simulink model "Project_Final_4_new"  (R2023b)
settings: Solver=VariableStepAuto  StartTime=0.0  StopTime=10.0  RelTol=1e-3
undefined symbols (not defined in the file or in its folder): batData, carData, motorData
libraries: slpidlib x1
settings Model: Creator=stick  LastModifiedBy=stick
settings RTWCC: GPUComputeCapability=5.0

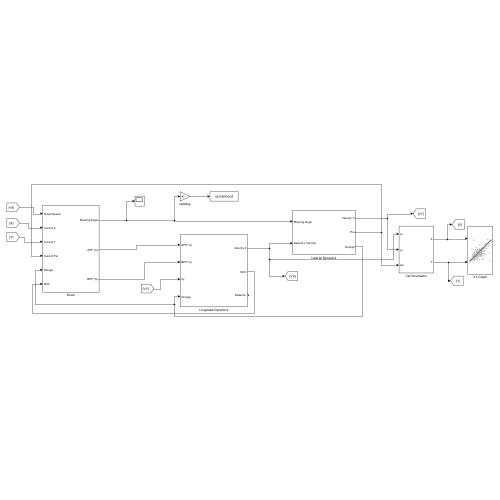
[thumbnail: Simulink's stored preview of the top-level diagram]
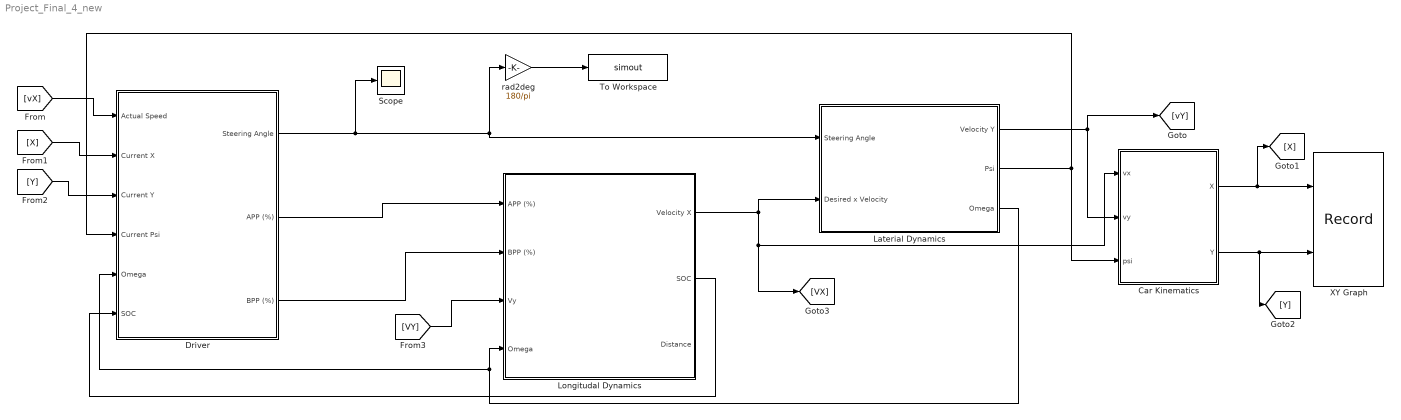
== system Project_Final_4_new ==
  Car Kinematics : Subsystem
  Driver : Subsystem
  Laterial Dynamics : Subsystem
  Longitudal Dynamics : Subsystem
  Scope : Scope
  To Workspace : ToWorkspace  VariableName=simout  SaveFormat=Timeseries  SampleTime=-1
  XY Graph : Record  FileSettingsInternal="{\"entries\":[{\"content\":{\"excelSettings\":{\"content\":{},\"type\":\"Streamout.ExcelSettings\"}},\"type\":\"Streamout.FileSettingStorage\",\"uuid\":\"\"}],\"packageUris\":[\"http:\\/\\/schema.mathworks.com\\/mf0\\/streamout_blocks\\/R2020a\"],\"version\":\"1.0\"}"  Layout=[1 1]  SignalsInternal="{\"entries\":[{\"content\":{\"signals\":[{\"content\":{\"blockPath\":[],\"dimensions\":[1],\"domain\":\"\",\"lineColor\":\"#d95319\",\"plots\":[ 1 ],\"port\":1,\"signalID\":1,\"signalName\":\"Car Kinematics:1\"},\"type\":\"RecordBlkView.Signal\",\"uuid\":\"\"},{\"content\":{\"blockPath\":[],\"dimensions\":[1],\"domain\":\"\",\"lineColor\":\"#edb120\",\"plots\":[ 1 ],\"port\":2,\"signalID\":2,\"signalName\":\"Car Kinematics:2\"},\"type\":\"RecordBlkView.Signal\",\"uuid\":\"\"}]},\"type\":\"RecordBlkView.InputSignals\",\"uuid\":\"\"}],\"packageUris\":[\"http:\\/\\/schema.mathworks.com\\/mf0\\/streamout_blocks\\/R2020a\"],\"version\":\"1.0\"}"  VisualizationBindings="{\"xyplotplugin\":{\"info\":[{\"series\":[{\"bindingParametersList\":[{\"parameter\":\"X-Axis\",\"signalID\":1,\"signalName\":\"Car Kinematics:1\"},{\"parameter\":\"Y-Axis\",\"signalID\":2,\"signalName\":\"Car Kinematics:2\"}],\"seriesID\":0}],\"subplotID\":1}]}}"  CompatibilityTag=XY  st=-1
  rad2deg : Gain  Gain=180/pi
  wires:
  [VY] -> Longitudal Dynamics/3(Vy)
  Driver/2(APP (%)) -> Longitudal Dynamics/1(APP (%))
  Driver/3(BPP (%)) -> Longitudal Dynamics/2(BPP (%))
  Laterial Dynamics/1(Velocity Y) -> [vY], Car Kinematics/2(vy)
  Longitudal Dynamics/1(Velocity X) -> [VX], Car Kinematics/1(vx), Laterial Dynamics/2(Desired x Velocity)
  Laterial Dynamics/2(Psi) -> Driver/4(Current Psi), Car Kinematics/3(psi)
  Laterial Dynamics/3(Omega) -> Longitudal Dynamics/4(Omega), Driver/5(Omega)
  Longitudal Dynamics/2(SOC) -> Driver/6(SOC)
  Driver/1(Steering Angle) -> Scope/1, rad2deg/1, Laterial Dynamics/1(Steering Angle)
  Car Kinematics/1(X) -> [X], XY Graph/1
  Car Kinematics/2(Y) -> [Y], XY Graph/2
  rad2deg/1 -> To Workspace/1
  [vX] -> Driver/1(Actual Speed)
  [X] -> Driver/2(Current X)
  [Y] -> Driver/3(Current Y)

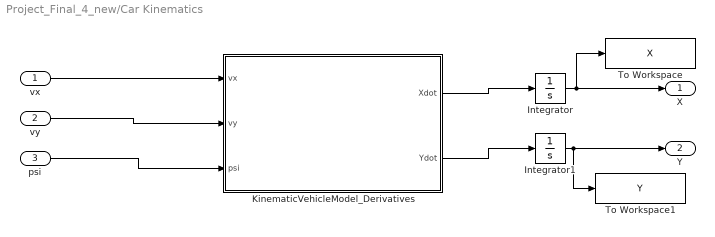
== system Project_Final_4_new/Car Kinematics ==
  vx : Inport
  vy : Inport  Port=2
  psi : Inport  Port=3
  Integrator : Integrator  InitialCondition=carData.init.X0
  Integrator1 : Integrator  InitialCondition=carData.init.Y0
  KinematicVehicleModel_Derivatives : MATLAB Function  TreatAsAtomicUnit=on
  To Workspace : ToWorkspace  VariableName=X  SaveFormat=Timeseries  SampleTime=-1
  To Workspace1 : ToWorkspace  VariableName=Y  SaveFormat=Timeseries  SampleTime=-1
  X : Outport
  Y : Outport  Port=2
  wires:
  Integrator1/1 -> To Workspace1/1, Y/1
  vy/1 -> KinematicVehicleModel_Derivatives/2(vy)
  vx/1 -> KinematicVehicleModel_Derivatives/1(vx)
  KinematicVehicleModel_Derivatives/2(Ydot) -> Integrator1/1
  psi/1 -> KinematicVehicleModel_Derivatives/3(psi)
  Integrator/1 -> To Workspace/1, X/1
  KinematicVehicleModel_Derivatives/1(Xdot) -> Integrator/1

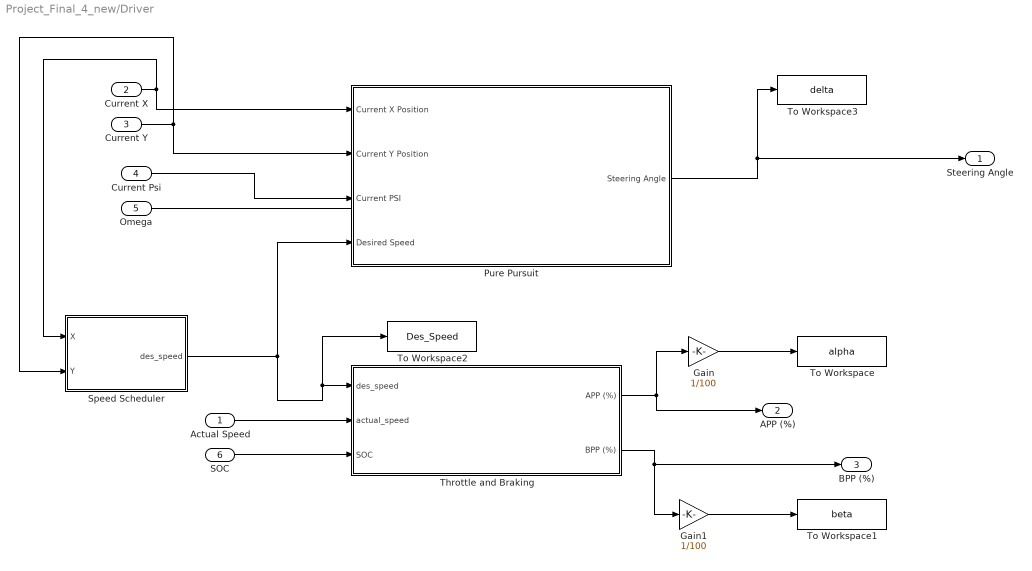
== system Project_Final_4_new/Driver ==
  Actual Speed : Inport
  Current X : Inport  Port=2
  Current Y : Inport  Port=3
  Current Psi : Inport  Port=4
  Omega : Inport  Port=5
  SOC : Inport  Port=6
  Gain : Gain  Gain=1/100
  Gain1 : Gain  Gain=1/100
  Pure Pursuit : Subsystem
  Speed Scheduler : MATLAB Function  TreatAsAtomicUnit=on
  Throttle and Braking : Subsystem
  To Workspace : ToWorkspace  VariableName=alpha  SaveFormat=Timeseries  SampleTime=-1
  To Workspace1 : ToWorkspace  VariableName=beta  SaveFormat=Timeseries  SampleTime=-1
  To Workspace2 : ToWorkspace  VariableName=Des_Speed  SaveFormat=Timeseries  SampleTime=-1
  To Workspace3 : ToWorkspace  VariableName=delta  SaveFormat=Timeseries  SampleTime=-1
  Steering Angle : Outport
  APP (%) : Outport  Port=2
  BPP (%) : Outport  Port=3
  wires:
  Throttle and Braking/1(APP (%)) -> APP (%)/1, Gain/1
  Throttle and Braking/2(BPP (%)) -> BPP (%)/1, Gain1/1
  Speed Scheduler/1(des_speed) -> To Workspace2/1, Throttle and Braking/1(des_speed), Pure Pursuit/4(Desired Speed)
  Pure Pursuit/1(Steering Angle) -> Steering Angle/1, To Workspace3/1
  Gain/1 -> To Workspace/1
  Gain1/1 -> To Workspace1/1
  Actual Speed/1 -> Throttle and Braking/2(actual_speed)
  SOC/1 -> Throttle and Braking/3(SOC)
  Current Psi/1 -> Pure Pursuit/3(Current PSI)
  Omega/1 -> ?
  Current X/1 -> Speed Scheduler/1(X), Pure Pursuit/1(Current X Position)
  Current Y/1 -> Speed Scheduler/2(Y), Pure Pursuit/2(Current Y Position)

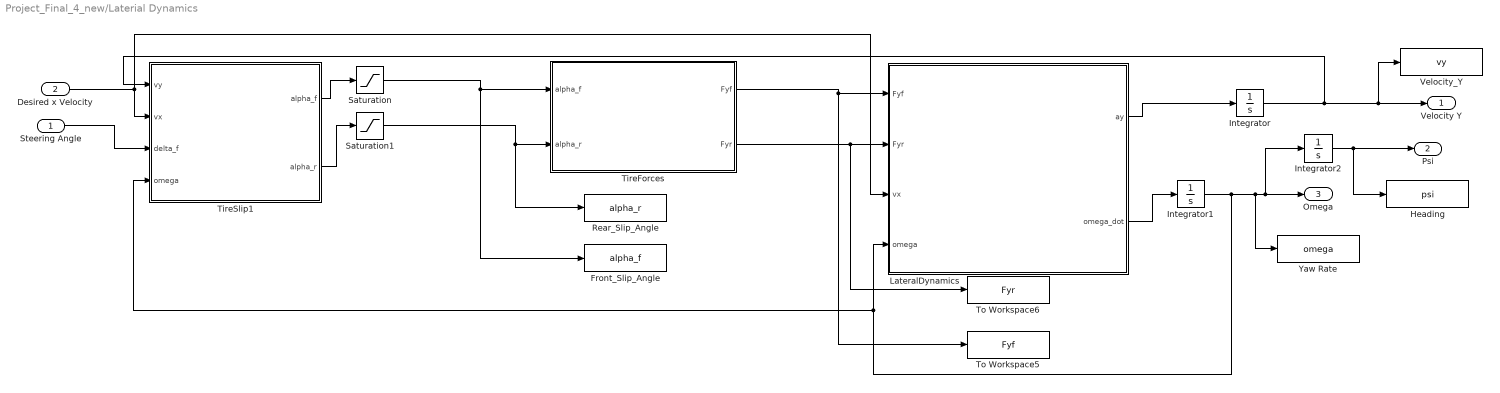
== system Project_Final_4_new/Laterial Dynamics ==
  Steering Angle : Inport
  Desired x Velocity : Inport  Port=2
  Front_Slip_Angle : ToWorkspace  VariableName=alpha_f  SaveFormat=Timeseries  SampleTime=-1
  Heading : ToWorkspace  VariableName=psi  SaveFormat=Timeseries  SampleTime=-1
  Integrator : Integrator  InitialCondition=carData.init.vy0
  Integrator1 : Integrator  InitialCondition=carData.init.omega0
  Integrator2 : Integrator  InitialCondition=carData.init.psi0  WrappedStateUpperValue=2*pi  WrappedStateLowerValue=0
  LateralDynamics : MATLAB Function  TreatAsAtomicUnit=on
  Rear_Slip_Angle : ToWorkspace  VariableName=alpha_r  SaveFormat=Timeseries  SampleTime=-1
  Saturation : Saturate  UpperLimit=carData.maxAlpha  LowerLimit=-carData.maxAlpha
  Saturation1 : Saturate  UpperLimit=carData.maxAlpha  LowerLimit=-carData.maxAlpha
  TireForces : MATLAB Function  TreatAsAtomicUnit=on
  TireSlip1 : MATLAB Function  TreatAsAtomicUnit=on
  To Workspace5 : ToWorkspace  VariableName=Fyf  SaveFormat=Timeseries  SampleTime=-1
  To Workspace6 : ToWorkspace  VariableName=Fyr  SaveFormat=Timeseries  SampleTime=-1
  Velocity_Y : ToWorkspace  VariableName=vy  SaveFormat=Timeseries  SampleTime=-1
  Yaw Rate : ToWorkspace  VariableName=omega  SaveFormat=Timeseries  SampleTime=-1
  Velocity Y : Outport
  Psi : Outport  Port=2
  Omega : Outport  Port=3
  wires:
  TireSlip1/2(alpha_r) -> Saturation1/1
  Integrator1/1 -> Omega/1, Integrator2/1, Yaw Rate/1, LateralDynamics/4(omega), TireSlip1/4(omega)
  LateralDynamics/1(ay) -> Integrator/1
  Saturation/1 -> Front_Slip_Angle/1, TireForces/1(alpha_f)
  TireForces/2(Fyr) -> LateralDynamics/2(Fyr), To Workspace6/1
  Steering Angle/1 -> TireSlip1/3(delta_f)
  LateralDynamics/2(omega_dot) -> Integrator1/1
  Desired x Velocity/1 -> TireSlip1/2(vx), LateralDynamics/3(vx)
  TireSlip1/1(alpha_f) -> Saturation/1
  Integrator2/1 -> Psi/1, Heading/1
  TireForces/1(Fyf) -> LateralDynamics/1(Fyf), To Workspace5/1
  Integrator/1 -> TireSlip1/1(vy), Velocity Y/1, Velocity_Y/1
  Saturation1/1 -> TireForces/2(alpha_r), Rear_Slip_Angle/1

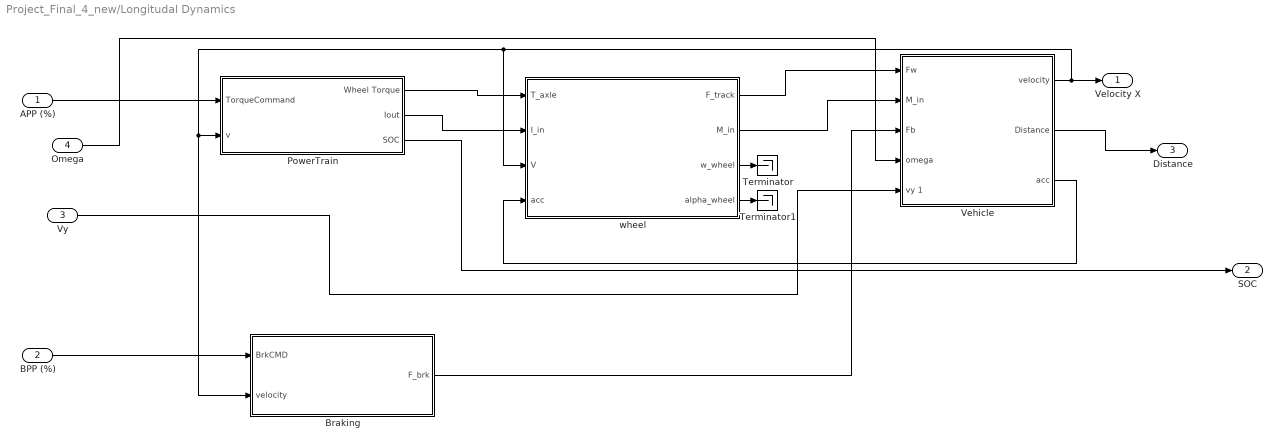
== system Project_Final_4_new/Longitudal Dynamics ==
  APP (%) : Inport
  BPP (%) : Inport  Port=2
  Vy : Inport  Port=3
  Omega : Inport  Port=4
  Braking : Subsystem
  PowerTrain : Subsystem
  Terminator : Terminator
  Terminator1 : Terminator
  Vehicle : Subsystem
  "wheel " : Subsystem
  Velocity X : Outport
  SOC : Outport  Port=2
  "Distance " : Outport  Port=3
  wires:
  Vehicle/1("velocity ") -> Velocity X/1, Braking/2("velocity "), PowerTrain/2(v), "wheel "/3(V)
  "wheel "/3(w_wheel) -> Terminator/1
  "wheel "/4(alpha_wheel) -> Terminator1/1
  APP (%)/1 -> PowerTrain/1(TorqueCommand)
  Vehicle/3(acc) -> "wheel "/4(acc)
  "wheel "/2(M_in) -> Vehicle/2("M_in ")
  "wheel "/1(F_track) -> Vehicle/1("Fw ")
  Vy/1 -> Vehicle/5(vy 1)
  Braking/1("F_brk ") -> Vehicle/3("Fb ")
  PowerTrain/2(Iout) -> "wheel "/2(I_in)
  PowerTrain/1(Wheel Torque) -> "wheel "/1(T_axle)
  Omega/1 -> Vehicle/4(omega)
  BPP (%)/1 -> Braking/1("BrkCMD ")
  PowerTrain/3(SOC) -> SOC/1
  Vehicle/2("Distance ") -> "Distance "/1

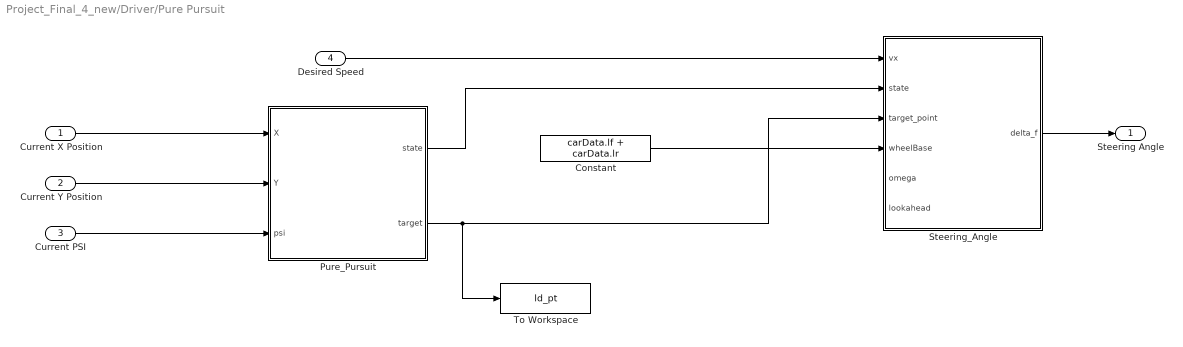
== system Project_Final_4_new/Driver/Pure Pursuit ==
  Current X Position : Inport
  Current Y Position : Inport  Port=2
  Current PSI : Inport  Port=3
  Desired Speed : Inport  Port=4
  Constant : Constant  Value=carData.lf + carData.lr
  Pure_Pursuit : MATLAB Function  TreatAsAtomicUnit=on
  Steering_Angle : MATLAB Function  TreatAsAtomicUnit=on
  To Workspace : ToWorkspace  VariableName=ld_pt  SaveFormat=Timeseries  SampleTime=-1
  Steering Angle : Outport
  wires:
  Constant/1 -> Steering_Angle/4(wheelBase)
  Steering_Angle/1(delta_f) -> Steering Angle/1
  Pure_Pursuit/2(target) -> Steering_Angle/3(target_point), To Workspace/1
  Pure_Pursuit/1(state) -> Steering_Angle/2(state)
  Desired Speed/1 -> Steering_Angle/1(vx)
  Current PSI/1 -> Pure_Pursuit/3(psi)
  Current Y Position/1 -> Pure_Pursuit/2(Y)
  Current X Position/1 -> Pure_Pursuit/1(X)

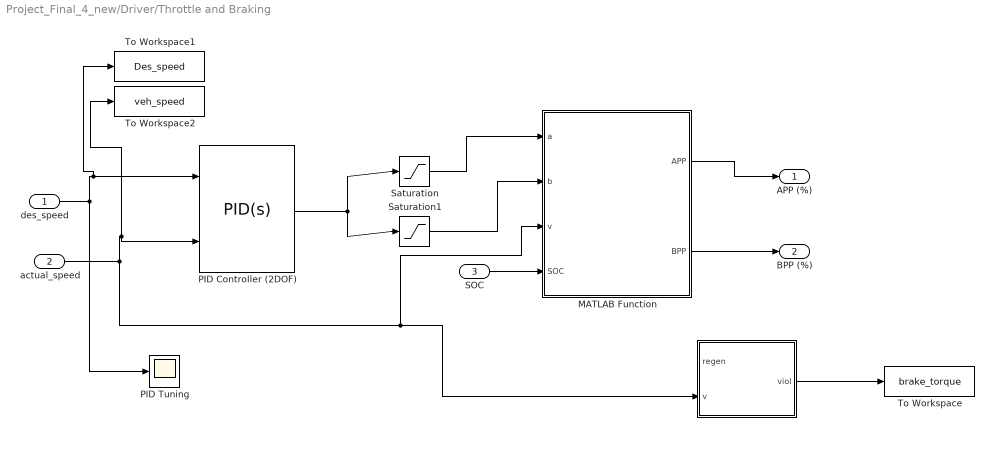
== system Project_Final_4_new/Driver/Throttle and Braking ==
  des_speed : Inport
  actual_speed : Inport  Port=2
  SOC : Inport  Port=3
  "  " : MATLAB Function  TreatAsAtomicUnit=on
  MATLAB Function : MATLAB Function  TreatAsAtomicUnit=on
  PID Controller (2DOF) : slpidlib/PID Controller (2DOF)  Controller=PID  Form=Parallel  TimeDomain=Continuous-time  UseExternalTs=off  SampleTime=-1  IntegratorMethod=Forward Euler  FilterMethod=Forward Euler  ControllerParametersSource=internal  P=1  I=1  UseKiTs=off  D=0  N=100  UseFilter=on  b=1  c=1  TunerSelectOption=Transfer Function Based (PID Tuner App)  InitialConditionSource=internal  InitialConditionForIntegrator=0  InitialConditionForFilter=0  DifferentiatorICPrevScaledInput=0  ExternalReset=none  TrackingMode=off  Kt=1  LimitOutput=off  SatLimitsSource=internal  UpperSaturationLimit=inf  LowerSaturationLimit=-inf  LinearizeAsGain=on  AntiWindupMode=none  Kb=1  LimitIntegrator=off  UpperIntegratorSaturationLimit=inf  LowerIntegratorSaturationLimit=-inf  POutMin=[]  POutMax=[]  IOutMin=[]  IOutMax=[]  DOutMin=[]  DOutMax=[]  NOutMin=[]  NOutMax=[]  bOutMin=[]  bOutMax=[]  cOutMin=[]  cOutMax=[]  SumOutMin=[]  SumOutMax=[]  SaturationOutMin=[]  SaturationOutMax=[]  PParamMin=[]  PParamMax=[]  IParamMin=[]  IParamMax=[]  DParamMin=[]  DParamMax=[]  NParamMin=[]  NParamMax=[]  bParamMin=[]  bParamMax=[]  cParamMin=[]  cParamMax=[]  KbParamMin=[]  KbParamMax=[]  KtParamMin=[]  KtParamMax=[]  KbOutMin=[]  KbOutMax=[]  KtOutMin=[]  KtOutMax=[]  IntegratorOutMin=[]  IntegratorOutMax=[]  FilterOutMin=[]  FilterOutMax=[]  SumI1OutMin=[]  SumI1OutMax=[]  SumI2OutMin=[]  SumI2OutMax=[]  SumI3OutMin=[]  SumI3OutMax=[]  SumI4OutMin=[]  SumI4OutMax=[]  SumDOutMin=[]  SumDOutMax=[]  Sum1OutMin=[]  Sum1OutMax=[]  Sum2OutMin=[]  Sum2OutMax=[]  Sum3OutMin=[]  Sum3OutMax=[]  DifferentiatorOutMin=[]  DifferentiatorOutMax=[]  FilterDiffOutCoefMin=[]  FilterDiffOutCoefMax=[]  ReciprocalOutMin=[]  ReciprocalOutMax=[]  SumDenOutMin=[]  SumDenOutMax=[]  SumNumOutMin=[]  SumNumOutMax=[]  DivideOutMin=[]  DivideOutMax=[]  UdiffTsProdOutMin=[]  UdiffTsProdOutMax=[]  NTsProdOutMin=[]  NTsProdOutMax=[]  UintegralTsProdOutMin=[]  UintegralTsProdOutMax=[]  UngainTsProdOutMin=[]  UngainTsProdOutMax=[]  ClampingZeroOutDataTypeStr=Inherit: Inherit via back propagation  ClampingZeroOutMin=[]  ClampingZeroOutMax=[]  FilterDenConstantOutDataTypeStr=Inherit: Inherit via back propagation  FilterDenConstantOutMin=[]  FilterDenConstantOutMax=[]  PCopyOutDataTypeStr=Inherit: Inherit via back propagation  PCopyOutMin=[]  PCopyOutMax=[]  NCopyOutDataTypeStr=Inherit: Inherit via back propagation  NCopyOutMin=[]  NCopyOutMax=[]  IntegratorContinuousStateAttributes=''  IntegratorStateMustResolveToSignalObject=off  IntegratorRTWStateStorageClass=Auto  FilterContinuousStateAttributes=''  FilterStateMustResolveToSignalObject=off  FilterRTWStateStorageClass=Auto  ParallelPVariant=InternalParameters  IdealPVariant=Disabled  IVariant=InternalParameters  DVariant=InternalParameters  bVariant=InternalParameters  cVariant=InternalParameters  IntegratorVariant=Continuous  SatVariant=Disabled  AWVariant=Passthrough  PCopyVariant=Disabled  TRVariant=Disabled  FdbkBlocksVariant=Forward  IdealPFdbkVariant=Disabled  SatFdbkVariant=Disabled  DerivativeFilterVariant=ContFilter  NVariant=InternalParameters  NCopyVariant=Disabled  FilterICVariant=InternalICsFilter  IntegratorICVariant=InternalICs  ExternalResetVariant=Disabled  TRSumVariant=Passthrough  SumFdbkVariant=Disabled  SumVariant=Sum_PID  TsampFilterVariant=InternalTs  TsampNgainVariant=Passthrough  TsampIntegralVariant=Disabled_SignalSpec  ExternalSaturationOutDataTypeStr=Inherit: Same as second input
  PID Tuning : Scope
  Saturation : Saturate  UpperLimit=1  LowerLimit=0
  Saturation1 : Saturate  UpperLimit=0  LowerLimit=-1
  To Workspace : ToWorkspace  VariableName=brake_torque  SaveFormat=Timeseries  SampleTime=-1
  To Workspace1 : ToWorkspace  VariableName=Des_speed  SaveFormat=Timeseries  SampleTime=-1
  To Workspace2 : ToWorkspace  VariableName=veh_speed  SaveFormat=Timeseries  SampleTime=-1
  APP (%) : Outport
  BPP (%) : Outport  Port=2
  wires:
  des_speed/1 -> PID Tuning/1, To Workspace1/1, PID Controller (2DOF)/1
  PID Controller (2DOF)/1 -> Saturation1/1, Saturation/1
  "  "/1(viol) -> To Workspace/1
  actual_speed/1 -> MATLAB Function/3(v), "  "/2(v), To Workspace2/1, PID Controller (2DOF)/2
  SOC/1 -> MATLAB Function/4(SOC)
  MATLAB Function/2(BPP) -> BPP (%)/1
  MATLAB Function/1(APP) -> APP (%)/1
  Saturation/1 -> MATLAB Function/1(a)
  Saturation1/1 -> MATLAB Function/2(b)

== system Project_Final_4_new/Longitudal Dynamics/Braking ==
  "BrkCMD " : Inport
  "velocity " : Inport  Port=2
  Gain1 : Gain  Gain=1.09
  MATLAB Function : MATLAB Function  TreatAsAtomicUnit=on
  "F_brk " : Outport  VectorParamsAs1DForOutWhenUnconnected=off
  wires:
  "BrkCMD "/1 -> Gain1/1
  Gain1/1 -> MATLAB Function/1(u)
  MATLAB Function/1(y) -> "F_brk "/1
  "velocity "/1 -> MATLAB Function/2(v)

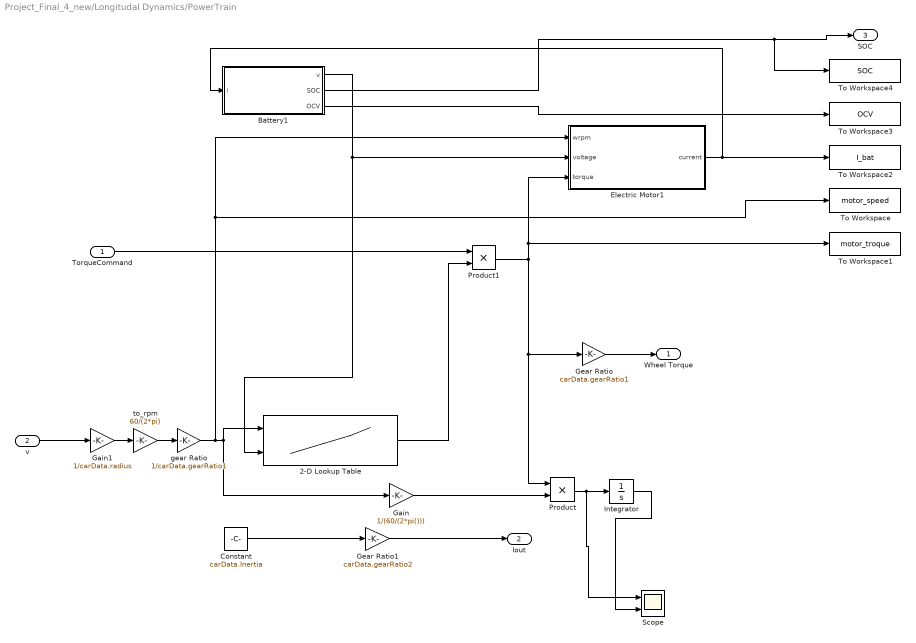
== system Project_Final_4_new/Longitudal Dynamics/PowerTrain ==
  TorqueCommand : Inport
  v : Inport  Port=2
  2-D Lookup Table : Lookup_n-D  BreakpointsForDimension1=motorData.vbus  BreakpointsForDimension2=motorData.rpm  Table=motorData.maxtorque  InternalRulePriority=Speed  RndMeth=Simplest
      settings: InputPortMap=u0,u1
  Battery1 : Subsystem
  Constant : Constant  Value=carData.Inertia
  Electric Motor1 : Subsystem
  Gain : Gain  Gain=1/(60/(2*pi()))
  Gain1 : Gain  Gain=1/carData.radius
  Gear Ratio : Gain  Gain=carData.gearRatio1
  Gear Ratio1 : Gain  Gain=carData.gearRatio2
  Integrator : Integrator
  Product : Product
  Product1 : Product
  Scope : Scope  NumInputPorts=2
  To Workspace : ToWorkspace  VariableName=motor_speed  SaveFormat=Structure With Time  SampleTime=-1
  To Workspace1 : ToWorkspace  VariableName=motor_troque  SaveFormat=Structure With Time  SampleTime=-1
  To Workspace2 : ToWorkspace  VariableName=I_bat  SaveFormat=Structure With Time  SampleTime=-1
  To Workspace3 : ToWorkspace  VariableName=OCV  SaveFormat=Structure With Time  SampleTime=-1
  To Workspace4 : ToWorkspace  VariableName=SOC  SaveFormat=Structure With Time  SampleTime=-1
  gear Ratio : Gain  Gain=1/carData.gearRatio1
  to_rpm : Gain  Gain=60/(2*pi)
  Wheel Torque : Outport
  Iout : Outport  Port=2
  SOC : Outport  Port=3
  wires:
  TorqueCommand/1 -> Product1/1
  Constant/1 -> Gear Ratio1/1
  v/1 -> Gain1/1
  Gain1/1 -> to_rpm/1
  2-D Lookup Table/1 -> Product1/2
  Product1/1 -> Product/1, Gear Ratio/1, Electric Motor1/3(torque), To Workspace1/1
  to_rpm/1 -> gear Ratio/1
  gear Ratio/1 -> Electric Motor1/1(wrpm), To Workspace/1, Gain/1, 2-D Lookup Table/1
  Gear Ratio/1 -> Wheel Torque/1
  Product/1 -> Scope/1, Integrator/1
  Integrator/1 -> Scope/2
  Gain/1 -> Product/2
  Battery1/1(v) -> 2-D Lookup Table/2, Electric Motor1/2(voltage)
  Electric Motor1/1(current) -> To Workspace2/1, Battery1/1(i)
  Gear Ratio1/1 -> Iout/1
  Battery1/2(SOC) -> To Workspace4/1, SOC/1
  Battery1/3(OCV) -> To Workspace3/1

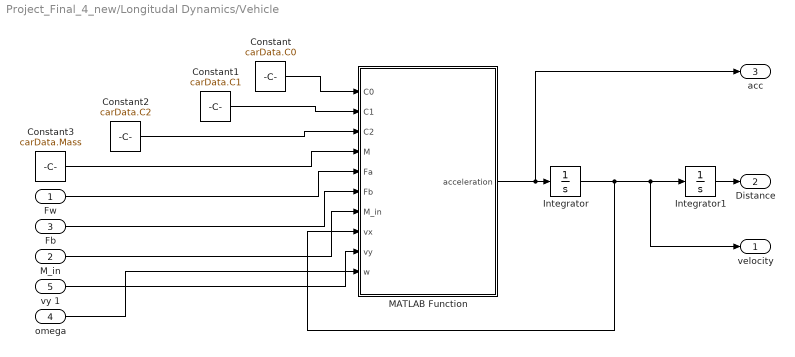
== system Project_Final_4_new/Longitudal Dynamics/Vehicle ==
  "Fw " : Inport
  "M_in " : Inport  Port=2
  "Fb " : Inport  Port=3
  omega : Inport  Port=4
  vy 1 : Inport  Port=5
  Constant : Constant  Value=carData.C0
  Constant1 : Constant  Value=carData.C1
  Constant2 : Constant  Value=carData.C2
  Constant3 : Constant  Value=carData.Mass
  Integrator : Integrator  LimitOutput=on  LowerSaturationLimit=0
  Integrator1 : Integrator
  MATLAB Function : MATLAB Function  TreatAsAtomicUnit=on
  "velocity " : Outport  VectorParamsAs1DForOutWhenUnconnected=off
  "Distance " : Outport  Port=2  VectorParamsAs1DForOutWhenUnconnected=off
  acc : Outport  Port=3
  wires:
  Constant1/1 -> MATLAB Function/2(C1)
  Constant/1 -> MATLAB Function/1(C0)
  MATLAB Function/1(acceleration) -> acc/1, Integrator/1
  Constant2/1 -> MATLAB Function/3(C2)
  Constant3/1 -> MATLAB Function/4(M)
  "Fw "/1 -> MATLAB Function/5(Fa)
  "Fb "/1 -> MATLAB Function/6(Fb)
  Integrator/1 -> MATLAB Function/8(vx), "velocity "/1, Integrator1/1
  Integrator1/1 -> "Distance "/1
  "M_in "/1 -> MATLAB Function/7(M_in)
  omega/1 -> MATLAB Function/10(w)
  vy 1/1 -> MATLAB Function/9(vy)

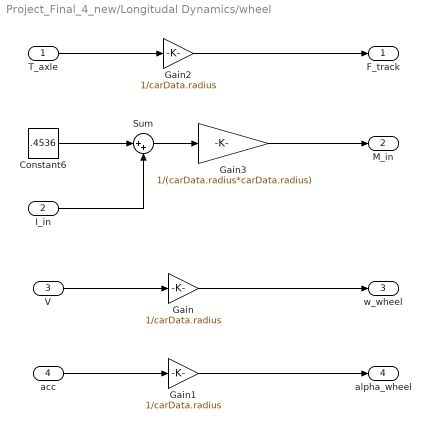
== system Project_Final_4_new/Longitudal Dynamics/wheel  ==
  T_axle : Inport
  I_in : Inport  Port=2
  V : Inport  Port=3
  acc : Inport  Port=4
  Constant6 : Constant  Value=.4536
  Gain : Gain  Gain=1/carData.radius
  Gain1 : Gain  Gain=1/carData.radius
  Gain2 : Gain  Gain=1/carData.radius
  Gain3 : Gain  Gain=1/(carData.radius*carData.radius)
  Sum : Sum  Inputs=|++
  F_track : Outport
  M_in : Outport  Port=2
  w_wheel : Outport  Port=3
  alpha_wheel : Outport  Port=4
  wires:
  Gain/1 -> w_wheel/1
  V/1 -> Gain/1
  acc/1 -> Gain1/1
  Gain1/1 -> alpha_wheel/1
  T_axle/1 -> Gain2/1
  Gain2/1 -> F_track/1
  Gain3/1 -> M_in/1
  Constant6/1 -> Sum/1
  I_in/1 -> Sum/2
  Sum/1 -> Gain3/1

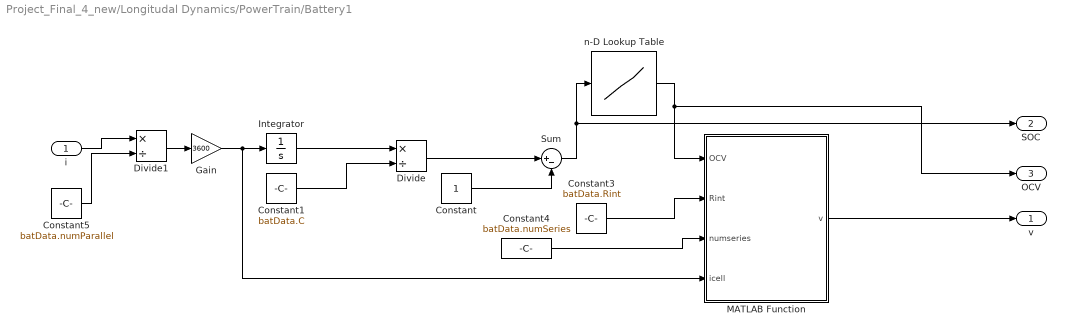
== system Project_Final_4_new/Longitudal Dynamics/PowerTrain/Battery1 ==
  i : Inport
  Constant : Constant
  Constant1 : Constant  Value=batData.C
  Constant3 : Constant  Value=batData.Rint
  Constant4 : Constant  Value=batData.numSeries
  Constant5 : Constant  Value=batData.numParallel
  Divide : Product  Inputs=*/
  Divide1 : Product  Inputs=*/
  Gain : Gain  Gain=3600
  Integrator : Integrator
  MATLAB Function : MATLAB Function  TreatAsAtomicUnit=on
  Sum : Sum  Inputs=|+-
  n-D Lookup Table : Lookup_n-D  NumberOfTableDimensions=1  BreakpointsForDimension1=batData.SOC  BreakpointsForDimension3=[5, 7]  Table=batData.OCV  InternalRulePriority=Speed  RndMeth=Simplest
  v : Outport
  SOC : Outport  Port=2
  OCV : Outport  Port=3
  wires:
  Constant/1 -> Sum/2
  Integrator/1 -> Divide/1
  Divide/1 -> Sum/1
  Constant1/1 -> Divide/2
  MATLAB Function/1(v) -> v/1
  Constant4/1 -> MATLAB Function/3(numseries)
  Divide1/1 -> Gain/1
  Constant5/1 -> Divide1/2
  i/1 -> Divide1/1
  Constant3/1 -> MATLAB Function/2(Rint)
  Sum/1 -> SOC/1, n-D Lookup Table/1
  n-D Lookup Table/1 -> OCV/1, MATLAB Function/1(OCV)
  Gain/1 -> MATLAB Function/4(icell), Integrator/1

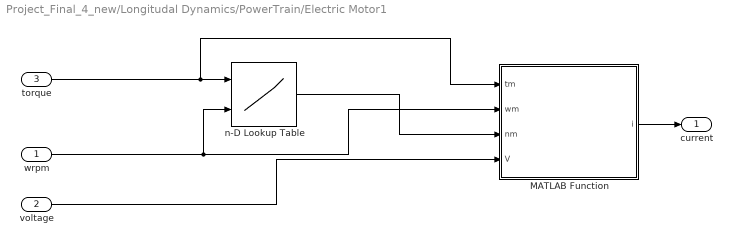
== system Project_Final_4_new/Longitudal Dynamics/PowerTrain/Electric Motor1 ==
  wrpm : Inport
  voltage : Inport  Port=2
  torque : Inport  Port=3
  MATLAB Function : MATLAB Function  TreatAsAtomicUnit=on
  n-D Lookup Table : Lookup_n-D  BreakpointsForDimension1=motorData.eta_torque  BreakpointsForDimension2=motorData.eta_speed  BreakpointsForDimension3=[5, 7]  Table=motorData.eta_val  InternalRulePriority=Speed  RndMeth=Simplest
      settings: InputPortMap=u0,u1
  current : Outport
  wires:
  torque/1 -> MATLAB Function/1(tm), n-D Lookup Table/1
  wrpm/1 -> MATLAB Function/2(wm), n-D Lookup Table/2
  n-D Lookup Table/1 -> MATLAB Function/3(nm)
  MATLAB Function/1(i) -> current/1
  voltage/1 -> MATLAB Function/4(V)

== matlab function Project_Final_4_new/Driver/Pure Pursuit/Pure_Pursuit ==
  data: state output; target output; X input; Y input; psi input
function [state,target] = fcn(X,Y, psi)

% creating a racetrack
% variables

x_i = [0];
y_i = [0];
x_o = [0];
x_p =[0];
y_p = [7.5];
y_o = [15];
radius = 200;
radius2 = 185;
center_right = [900,-200];
center_left = [0,-200];
theta = linspace(0,pi,1000);

% loop to obtain all values

for i = 1:900;
    j_i = 0;
    j_o = 7.5;
    x_p = [x_p, i];
    y_p = [y_p,j_i];
    x_i = [x_i, i];
    x_o = [x_o,i];
    y_o = [y_o,j_o];
    y_i = [y_i,j_i];
end

for i = 1:length(theta);
    x_o = [x_o, center_right(1)+radius*sin(theta(i))];
    x_i = [x_i, center_right(1)+radius2*sin(theta(i))];
    x_p = [x_p, center_right(1)+radius2*sin(theta(i))];
    y_p = [y_p, 15 + center_right(2)+radius*cos(theta(i))];
    y_o = [y_o, 15 + center_right(2)+radius*cos(theta(i))];
    y_i = [y_i, 15 + center_right(2)+radius2*cos(theta(i))];
end 

for i = 1:900;
    x_o = [x_o,900-i];
    x_i = [x_i,900-i];
    x_p = [x_p, 900-i];
    y_p = [y_p,-377.5];
    y_o = [y_o, -385];
    y_i = [y_i,-370];
end 

for i = 1:length(theta);
    x_o = [x_o, center_left(1)-radius*sin(theta(i))];
    x_i = [x_i, center_left(1)-radius2*sin(theta(i))];
    x_p = [x_p, center_left(1)-radius2*sin(theta(i))];
    y_p = [y_p, 15 + center_left(2)-radius*cos(theta(i))];
    y_o = [y_o, 15 + center_left(2)-radius*cos(theta(i))];
    y_i = [y_i, 15 + center_left(2)-radius2*cos(theta(i))];
end

waypoints_x = x_p;
waypoints_y = y_p;

% plotting racetrack
%plot(x_i, y_i)
%axis([-100 1000 -400 25])
%hold on
%plot(x_o,y_o)
%hold off

% code for plotting animated moving car
%variables for finding path to plot

x_p = [0];
y_p = [];
center_rightpath = [0,-192.5];
center_leftpath = [900,-192.5];
radius_path = -192.5; 

for i = 1:900;
    x_p = [x_p, i];
    y_p = [y_p,7.5];
end

for i = 1:length(theta);
    x_p = [x_p, center_leftpath(1)-radius_path*sin(theta(i))];
    y_p = [y_p, 7.5 + center_leftpath(2)-radius_path*cos(theta(i))];
end 

for i = 1:900;
    x_p = [x_p,900-i];
    y_p = [y_p,-377.5];
end 

for i = 1:length(theta);
    x_p = [x_p, center_rightpath(1)+radius_path*sin(theta(i))];
    y_p = [y_p, 7.5 + center_rightpath(2)+radius_path*cos(theta(i))];

end   
waypoints_y;
waypoints_x;

dist = zeros(1, numel(waypoints_x));

for i = 1:numel(waypoints_x)
    dist(i) = sqrt((waypoints_x(i) - X)^2 + (waypoints_y(i) - Y)^2);

end

[~, index] = min(dist);

target_psi = atan2(waypoints_y(index) - Y, waypoints_x(index) - X);


state =[X,Y,psi];

target = [waypoints_x(index), waypoints_y(index), target_psi];

== matlab function Project_Final_4_new/Driver/Pure Pursuit/Steering_Angle ==
  data: vx input; delta_f output; state input; target_point input; wheelBase input; omega input; lookahead input

function delta_f = latControl(vx, state, target_point, wheelBase, omega, lookahead)

current_X = state(1);
current_Y = state(2);
current_psi = state(3);

targ_X = target_point(1);
targ_Y = target_point(2);
tar_psi = target_point(3);

alpha = atan2(targ_Y-current_Y,targ_X - current_X)-current_psi;
psi_dot_d = (2*wheelbase*sin(alpha))/lookahead;
delta_f = atan(psi_dot_d);

== matlab function Project_Final_4_new/Driver/Throttle and Braking/MATLAB Function ==
  data: a input; b input; APP output; v input; SOC input; BPP output
function [APP,BPP] = fcn(a,b,v, SOC)
v = v;
SOC = SOC;
if a>0
    APP=a;
    BPP=0;
elseif b<0
    APP=0;
    BPP=b;
else
    APP=0;
    BPP=0;
end

== matlab function Project_Final_4_new/Laterial Dynamics/TireSlip1 ==
  data: vy input; alpha_f output; vx input; delta_f input; omega input; alpha_r output
function [alpha_f, alpha_r] = fnc(vy, vx, delta_f, omega)

    if abs(vx) > 0.1
        alpha_f = delta_f - (vy + omega *1) / vx;
        alpha_r = - (vy - omega * 1.5) / vx;
    else
        alpha_f = 0;
        alpha_r = 0;
    end

end

== matlab function Project_Final_4_new/Laterial Dynamics/LateralDynamics ==
  data: Fyf input; ay output; Fyr input; vx input; omega input; omega_dot output
function [ay, omega_dot] = fcn(Fyf, Fyr, vx, omega)

    Fy = Fyf + Fyr;
    ay = Fy / 1000 - omega * vx;

    M = Fyf * 1.5 - Fyr * 1;
    omega_dot = M / 1600;

end

== matlab function Project_Final_4_new/Longitudal Dynamics/PowerTrain/Electric Motor1/MATLAB Function ==
  data: tm input; i output; wm input; nm input; V input
function i = fcn(tm,wm,nm,V)

i = (tm*wm*(nm^((tm*wm)/(abs(tm*wm)+0.001)))) / V;

== matlab function Project_Final_4_new/Car Kinematics/KinematicVehicleModel_Derivatives ==
  data: vx input; Xdot output; vy input; psi input; Ydot output
function [Xdot, Ydot] = fcn(vx, vy, psi)
    temp = TF(psi) * [vx;vy];
    Xdot = temp(1);
    Ydot = temp(2);
end

function y = TF(psi)
    y = [cos(psi), -sin(psi); sin(psi), cos(psi)];
end

== matlab function Project_Final_4_new/Longitudal Dynamics/Braking/MATLAB Function ==
  data: u input; y output; v input
function y = fcn(u,v)
y = u * v/(abs(v)+0.001);

== matlab function Project_Final_4_new/Longitudal Dynamics/PowerTrain/Battery1/MATLAB Function ==
  data: v output; OCV input; Rint input; numseries input; icell input
function v = fcn(OCV, Rint, numseries, icell)

v = numseries * (OCV - Rint * icell) ;

== matlab function Project_Final_4_new/Laterial Dynamics/TireForces ==
  data: alpha_f input; Fyf output; alpha_r input; Fyr output
function [Fyf, Fyr] = fcn(alpha_f, alpha_r)

    Fyf = min((40000*1/180*pi), 40000 * alpha_f);
    Fyr = min((40000*1/180*pi), 40000 * alpha_r);

end

== matlab function Project_Final_4_new/Driver/Throttle and Braking/   ==
  data: regen input; viol output; v input
function viol = fcn(regen,v)
    if v < (5*(1600/3600));
        regen_vio = 0;
        if regen == regen_vio
            viol = 0;
        else
            viol = 1;
        end
    elseif v == (25*1600/3600)
        regen_vio = 0.95;
        if regen == regen_vio
            viol = 0;
        else
            viol = 1;
        end
    elseif v > (25*1600/3600)
        regen_vio = 0.95;
        if regen == regen_vio
            viol = 0;
        else
            viol = 1;
        end
    else 
        regen_vio = (0.95/20)*v;
        if regen ==regen_vio
            viol = 0;
        else 
            viol = 1;
        end
    end
end

== matlab function Project_Final_4_new/Longitudal Dynamics/Vehicle/MATLAB Function ==
  data: C0 input; acceleration output; C1 input; C2 input; M input; Fa input; Fb input; M_in input; vx input; vy input; w input
function acceleration   = vehicle(C0,C1,C2,M,Fa,Fb,M_in, vx, vy, w)

acceleration = (((Fa-Fb))-(C0+ C1*vx + C2*(vx)^2 + 9.8*M + vy*w))/(M+M_in);

== matlab function Project_Final_4_new/Driver/Speed Scheduler ==
  data: X input; des_speed output; Y input
function des_speed = fcn(X,Y)

des_speed = 40;
